simulink model "Copy_of_simu"  (R2017a)
settings: Solver=VariableStepAuto  StartTime=0.0  StopTime=10  RelTol=1e-3  EnableMultiTasking=on
values from neighbouring files (symbols this model uses):
  th1_0 = pi/3    (= 1.0471975512)    [projeeeeetttt2.m]
  th2_0 = pi/3    (= 1.0471975512)    [projeeeeetttt2.m]
  theta_0 = pi/3    (= 1.0471975512)    [projeeeeetttt2.m]
  Xd = 2.2    [projeeeeetttt2.m]
  Xe0 = Xr0 + l1*cos(theta_0+th1_0) + l2*cos(theta_0+th1_0+th2_0)    [projeeeeetttt2.m]
  Yd = 0.7    [projeeeeetttt2.m]
  Ye0 = Yr0 + l1*sin(theta_0+th1_0) + l2*sin(theta_0+th1_0+th2_0)    [projeeeeetttt2.m]
settings Model: Creator=max.sonzogni  LastModifiedBy=Max
settings DataIOCC: LimitDataPoints=on
settings OptimizationCC: LifeSpan=inf
settings DebuggingCC: AllowSymbolicDim=off  SFUnexpectedBacktrackingDiag=warning  SFNoUnconditionalDefaultTransitionDiag=warning  SFExecutionAtInitializationDiag=none
settings ModelReferenceCC: PropagateSignalLabelsOutOfModel=off
settings GRTTargetCC: TargetLangStandard=C89/C90 (ANSI)
settings ConfigComp: CovMetricSettings=dw  CovHtmlReporting=on  CovSaveCumulativeToWorkspaceVar=on  CovSaveSingleToWorkspaceVar=on  CovExternalEMLEnable=off

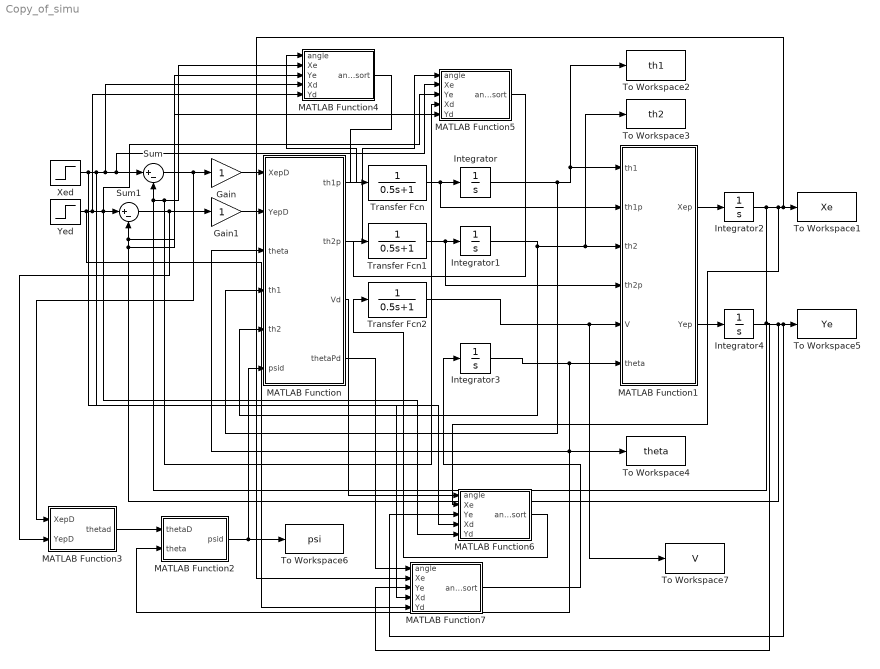
== system Copy_of_simu ==
  Gain : Gain
  Gain1 : Gain
  Integrator : Integrator  InitialCondition=th1_0
  Integrator1 : Integrator  InitialCondition=th2_0
  Integrator2 : Integrator  InitialCondition=Xe0
  Integrator3 : Integrator  InitialCondition=theta_0
  Integrator4 : Integrator  InitialCondition=Ye0
  MATLAB Function : MATLAB Function  TreatAsAtomicUnit=on
  MATLAB Function1 : MATLAB Function  TreatAsAtomicUnit=on
  MATLAB Function2 : MATLAB Function  TreatAsAtomicUnit=on
  MATLAB Function3 : MATLAB Function  TreatAsAtomicUnit=on
  MATLAB Function4 : MATLAB Function  TreatAsAtomicUnit=on
  MATLAB Function5 : MATLAB Function  TreatAsAtomicUnit=on
  MATLAB Function6 : MATLAB Function  TreatAsAtomicUnit=on
  MATLAB Function7 : MATLAB Function  TreatAsAtomicUnit=on
  Sum : Sum  Inputs=|+-
  Sum1 : Sum  Inputs=|+-
  To Workspace1 : ToWorkspace  VariableName=Xe  SampleTime=-1
  To Workspace2 : ToWorkspace  VariableName=th1  SampleTime=-1
  To Workspace3 : ToWorkspace  VariableName=th2  SampleTime=-1
  To Workspace4 : ToWorkspace  VariableName=theta  SampleTime=-1
  To Workspace5 : ToWorkspace  VariableName=Ye  SampleTime=-1
  To Workspace6 : ToWorkspace  VariableName=psi  SampleTime=-1
  To Workspace7 : ToWorkspace  VariableName=V  SampleTime=-1
  Transfer Fcn : TransferFcn  Denominator=[0.5 1]
  Transfer Fcn1 : TransferFcn  Denominator=[0.5 1]
  Transfer Fcn2 : TransferFcn  Denominator=[0.5 1]
  "Xed " : Step  Before=Xd  After=Xd  SampleTime=0
  "Yed " : Step  Before=Yd  After=Yd  SampleTime=0
  wires:
  "Xed "/1 -> MATLAB Function6/4(Xd), MATLAB Function7/4(Xd), MATLAB Function4/4(Xd), MATLAB Function5/2(Xe), Sum/1
  "Yed "/1 -> MATLAB Function7/5(Yd), MATLAB Function4/5(Yd), MATLAB Function6/5(Yd), MATLAB Function5/3(Ye), Sum1/1
  Transfer Fcn/1 -> MATLAB Function1/2(th1p), Integrator/1
  Transfer Fcn1/1 -> Integrator1/1, MATLAB Function1/4(th2p)
  Integrator1/1 -> To Workspace3/1, MATLAB Function1/3(th2), MATLAB Function/5(th2)
  Integrator3/1 -> MATLAB Function1/6(theta), MATLAB Function2/2(theta), MATLAB Function/3(theta), To Workspace4/1
  Integrator/1 -> MATLAB Function/4(th1), To Workspace2/1, MATLAB Function1/1(th1)
  Sum/1 -> Gain/1, MATLAB Function3/1(XepD)
  Sum1/1 -> Gain1/1, MATLAB Function3/2(YepD)
  MATLAB Function3/1(thetad) -> MATLAB Function2/1(thetaD)
  MATLAB Function2/1(psid) -> To Workspace6/1, MATLAB Function/6(psid)
  Transfer Fcn2/1 -> To Workspace7/1, MATLAB Function1/5(V)
  MATLAB Function1/1(Xep) -> Integrator2/1
  MATLAB Function1/2(Yep) -> Integrator4/1
  Integrator2/1 -> MATLAB Function6/2(Xe), MATLAB Function7/2(Xe), To Workspace1/1, MATLAB Function7/3(Ye), MATLAB Function5/4(Xd), MATLAB Function4/2(Xe), Sum/2
  Gain/1 -> MATLAB Function/1(XepD)
  Gain1/1 -> MATLAB Function/2(YepD)
  MATLAB Function/1(th1p) -> MATLAB Function4/1(angle)
  MATLAB Function4/1(angle_sort) -> Transfer Fcn/1
  MATLAB Function/2(th2p) -> MATLAB Function5/1(angle)
  MATLAB Function5/1(angle_sort) -> Transfer Fcn1/1
  Integrator4/1 -> MATLAB Function6/3(Ye), To Workspace5/1, MATLAB Function4/3(Ye), MATLAB Function5/5(Yd), Sum1/2
  MATLAB Function6/1(angle_sort) -> Transfer Fcn2/1
  MATLAB Function/3(Vd) -> MATLAB Function6/1(angle)
  MATLAB Function/4(thetaPd) -> MATLAB Function7/1(angle)
  MATLAB Function7/1(angle_sort) -> Integrator3/1

== matlab function Copy_of_simu/MATLAB Function1 ==
  data: th1 input; th1p input; Xep output; th2 input; th2p input; V input; theta input; Yep output
function [Xep,Yep] = vehicule(th1, th1p,th2,th2p,V,theta)

l1 = 0.8;
l2 = 0.55;

Xep = (-l1*sin(theta+th1)-l2*sin(theta+th1+th2))*th1p + (-l2*sin(theta+th1+th2))*th2p + V*cos(theta);
Yep = (l1*cos(theta+th1)+l2*cos(theta+th1+th2))*th1p + (l2*cos(theta+th1+th2))*th2p + V*sin(theta);

end

== matlab function Copy_of_simu/MATLAB Function ==
  data: XepD input; th1p output; YepD input; theta input; th1 input; th2 input; psid input; th2p output; Vd output; thetaPd output
function [th1p,th2p,Vd,thetaPd] = controle(XepD,YepD,theta,th1,th2,psid)

D = 1;
l1 = 0.8;
l2 = 0.55;

Vd = sqrt(XepD^2+YepD^2);
thetaPd = Vd*tan(psid)/D;

A = [-l1*sin(theta+th1)-l2*sin(theta+th1+th2) -l2*sin(theta+th1+th2) cos(theta)
    l1*cos(theta+th1)+l2*cos(theta+th1+th2) l2*cos(theta+th1+th2) sin(theta)
    0 0 tan(psid)/D];

res = inv(A)*[XepD;YepD;thetaPd];
th1p = res(1); th2p = res(2);
end

== matlab function Copy_of_simu/MATLAB Function2 ==
  data: thetaD input; psid output; theta input
function psid = anglediff(thetaD,theta)

u = thetaD; v = theta;

if u<-pi
    u = mod(u,-pi);
end
if u>pi
    u = mod(u,pi);
end
if v<-pi
    v = mod(v,-pi);
end
if v>pi
    v = mod(v,pi);
end
y = u-v;
if y<-pi
    y = mod(y,-pi);
end
if y>pi
    y = mod(y,pi);
end

psid = y;

end

== matlab function Copy_of_simu/MATLAB Function3 ==
  data: XepD input; YepD input; thetad output
function thetad = fcn(XepD,YepD)

thetad = atan(YepD/XepD);
%thetad = atan2(YepD,XepD);

end

== matlab function Copy_of_simu/MATLAB Function4 ==
  data: angle input; angle_sort output; Xe input; Ye input; Xd input; Yd input
function angle_sort = fcn(angle,Xe,Ye,Xd,Yd)

l1 = 0.8;
l2 = 0.55;
dist = (Xe-Xd)^2+(Ye-Yd)^2;
if dist > l1^2+l2^2
    angle_sort = 0;
else
    angle_sort = angle;

end

== matlab function Copy_of_simu/MATLAB Function5 ==
  data: angle input; angle_sort output; Xe input; Ye input; Xd input; Yd input
function angle_sort = fcn(angle,Xe,Ye,Xd,Yd)

l1 = 0.8;
l2 = 0.55;
dist = (Xe-Xd)^2+(Ye-Yd)^2;
if dist > l1^2+l2^2
    angle_sort = 0;
else
    angle_sort = angle;

end

== matlab function Copy_of_simu/MATLAB Function6 ==
  data: angle input; angle_sort output; Xe input; Ye input; Xd input; Yd input
function angle_sort = fcn(angle,Xe,Ye,Xd,Yd)

l1 = 0.8;
l2 = 0.55;
dist = (Xe-Xd)^2+(Ye-Yd)^2;
if dist < l1^2+l2^2
    angle_sort = angle/10;
else
    angle_sort = angle;

end

== matlab function Copy_of_simu/MATLAB Function7 ==
  data: angle input; angle_sort output; Xe input; Ye input; Xd input; Yd input
function angle_sort = fcn(angle,Xe,Ye,Xd,Yd)

l1 = 0.8;
l2 = 0.55;
dist = (Xe-Xd)^2+(Ye-Yd)^2;
if dist < l1^2+l2^2
    angle_sort = angle/10;
else
    angle_sort = angle;

end
